simulink model "A1_AAI"  (R2020a)
settings: Solver=FixedStepAuto  StartTime=0.0  StopTime=10  FixedStep=1e-3  RelTol=1e-3  EnableMultiTasking=on
undefined symbols (not defined in the file): D0, D10, D11, D12, D13, D2, D4, D5, D6, D7, D8, D9, PTA0, PTA2, PTB23, PTB9, PTC16, PTC2, PTC3, PTC4, PTD0, PTD1, PTD2, PTD3
libraries: frdmk64flib x16
settings Model: ExtModeTrigDuration=5  Creator=Faisal  LastModifiedBy=Faisal
settings OptimizationCC: EnhancedBackFolding=on  PassReuseOutputArgsAs=Individual arguments  ZeroExternalMemoryAtStartup=off  ZeroInternalMemoryAtStartup=off  MaxStackSize=64  OptimizeBlockOrder=speed  DifferentSizesBufferReuse=on  OptimizationCustomize=off  EfficientTunableParamExpr=on
settings DebuggingCC: ParameterTunabilityLossMsg=error
settings HardwareCC: ProdBitPerPointer=32  ProdBitPerSizeT=32  ProdBitPerPtrDiffT=32  ProdLargestAtomicInteger=Long  ProdLargestAtomicFloat=Double  ProdWordSize=32  ProdHWDeviceType=ARM Compatible->ARM Cortex
settings SFSimCC: MATLABDynamicMemAlloc=off
settings RTWCC: SystemTargetFile=ert.tlc  HardwareBoard=NXP FRDM-K64F  TemplateMakefile=ert_default_tmf  Toolchain=GNU Tools for ARM Embedded Processors
settings CodeAppCC: ForceParamTrailComments=on  IgnoreCustomStorageClasses=off  OperatorAnnotations=on  SimulinkDataObjDesc=on  SFDataObjDesc=on  InsertBlockDesc=on

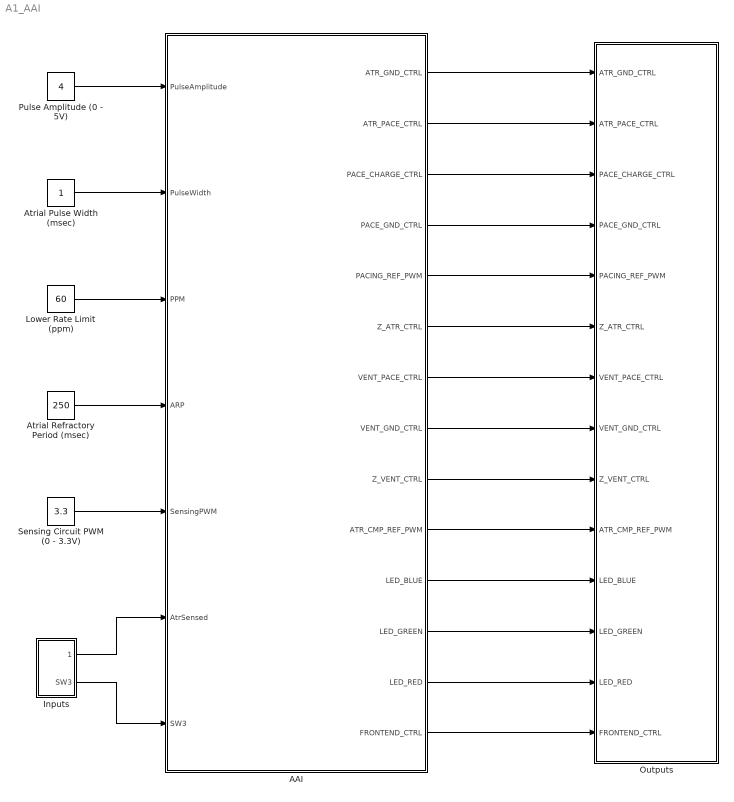
== system A1_AAI ==
  AAI : Stateflow chart  TreatAsAtomicUnit=on
  Atrial Pulse Width (msec) : Constant  OutDataTypeStr=double
  Atrial Refractory Period (msec) : Constant  Value=250  OutDataTypeStr=uint16
  Inputs : Subsystem
  Lower Rate Limit (ppm) : Constant  Value=60  OutDataTypeStr=uint16
  Outputs : Subsystem
  Pulse Amplitude (0 - 5V) : Constant  Value=4  OutDataTypeStr=double
  Sensing Circuit PWM (0 - 3.3V) : Constant  Value=3.3  OutDataTypeStr=double
  wires:
  Pulse Amplitude (0 - 5V)/1 -> AAI/1(PulseAmplitude)
  Atrial Pulse Width (msec)/1 -> AAI/2(PulseWidth)
  Lower Rate Limit (ppm)/1 -> AAI/3(PPM)
  Atrial Refractory Period (msec)/1 -> AAI/4(ARP)
  Sensing Circuit PWM (0 - 3.3V)/1 -> AAI/5(SensingPWM)
  AAI/1(ATR_GND_CTRL) -> Outputs/1(ATR_GND_CTRL)
  AAI/2(ATR_PACE_CTRL) -> Outputs/2(ATR_PACE_CTRL)
  AAI/3(PACE_CHARGE_CTRL) -> Outputs/3(PACE_CHARGE_CTRL)
  AAI/4(PACE_GND_CTRL) -> Outputs/4(PACE_GND_CTRL)
  AAI/5(PACING_REF_PWM) -> Outputs/5(PACING_REF_PWM)
  AAI/6(Z_ATR_CTRL) -> Outputs/6(Z_ATR_CTRL)
  AAI/7(VENT_PACE_CTRL) -> Outputs/7(VENT_PACE_CTRL)
  AAI/8(VENT_GND_CTRL) -> Outputs/8(VENT_GND_CTRL)
  AAI/9(Z_VENT_CTRL) -> Outputs/9(Z_VENT_CTRL)
  AAI/10(ATR_CMP_REF_PWM) -> Outputs/10(ATR_CMP_REF_PWM)
  AAI/11(LED_BLUE) -> Outputs/11(LED_BLUE)
  AAI/12(LED_GREEN) -> Outputs/12(LED_GREEN)
  AAI/13(LED_RED) -> Outputs/13(LED_RED)
  AAI/14(FRONTEND_CTRL) -> Outputs/14(FRONTEND_CTRL)
  Inputs/1(AtrSensed) -> AAI/6(AtrSensed)
  Inputs/2(SW3) -> AAI/7(SW3)

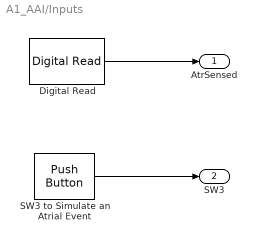
== system A1_AAI/Inputs ==
  Digital Read : frdmk64flib/Digital Read  Whichpin=PTC16 (D0)  SampleTime=-1
  SW3 to Simulate an Atrial Event : frdmk64flib/Push Button  Whichswitch=SW3  SampleTime1=-1
  AtrSensed : Outport
  SW3 : Outport  Port=2
  wires:
  Digital Read/1 -> AtrSensed/1
  SW3 to Simulate an Atrial Event/1 -> SW3/1

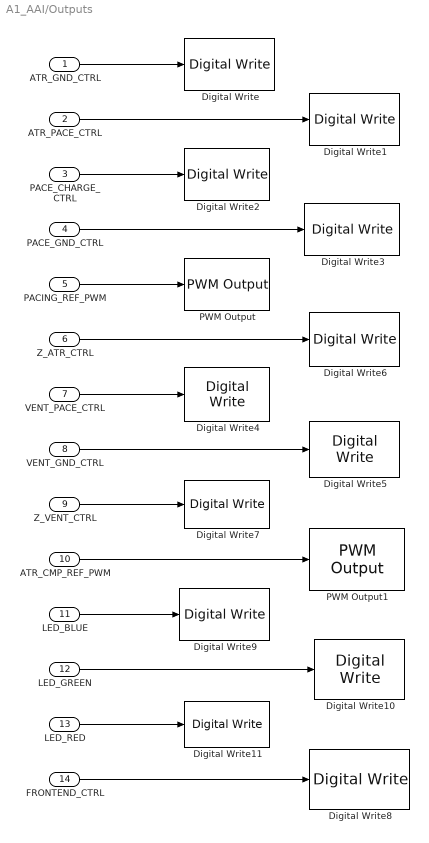
== system A1_AAI/Outputs ==
  ATR_GND_CTRL : Inport
  ATR_PACE_CTRL : Inport  Port=2
  PACE_CHARGE_CTRL : Inport  Port=3
  PACE_GND_CTRL : Inport  Port=4
  PACING_REF_PWM : Inport  Port=5
  Z_ATR_CTRL : Inport  Port=6
  VENT_PACE_CTRL : Inport  Port=7
  VENT_GND_CTRL : Inport  Port=8
  Z_VENT_CTRL : Inport  Port=9
  ATR_CMP_REF_PWM : Inport  Port=10
  LED_BLUE : Inport  Port=11
  LED_GREEN : Inport  Port=12
  LED_RED : Inport  Port=13
  FRONTEND_CTRL : Inport  Port=14
  Digital Write : frdmk64flib/Digital Write  Whichpin=PTD2 (D11)
  Digital Write1 : frdmk64flib/Digital Write  Whichpin=PTA0 (D8)
  Digital Write10 : frdmk64flib/Digital Write  Whichpin=GREEN_LED
  Digital Write11 : frdmk64flib/Digital Write  Whichpin=RED_LED
  Digital Write2 : frdmk64flib/Digital Write  Whichpin=PTB9 (D2)
  Digital Write3 : frdmk64flib/Digital Write  Whichpin=PTD0 (D10)
  Digital Write4 : frdmk64flib/Digital Write  Whichpin=PTC4 (D9)
  Digital Write5 : frdmk64flib/Digital Write  Whichpin=PTD3 (D12)
  Digital Write6 : frdmk64flib/Digital Write  Whichpin=PTB23 (D4)
  Digital Write7 : frdmk64flib/Digital Write  Whichpin=PTC3 (D7)
  Digital Write8 : frdmk64flib/Digital Write  Whichpin=PTD1 (D13)
  Digital Write9 : frdmk64flib/Digital Write  Whichpin=BLUE_LED
  PWM Output : frdmk64flib/PWM Output  Whichpin=PTA2 (D5)  InitialFrequency=2000  InitialDutyCycle=100
  PWM Output1 : frdmk64flib/PWM Output  Whichpin=PTC2 (D6)  InitialFrequency=2000  InitialDutyCycle=0
  wires:
  LED_BLUE/1 -> Digital Write9/1
  VENT_PACE_CTRL/1 -> Digital Write4/1
  Z_ATR_CTRL/1 -> Digital Write6/1
  LED_GREEN/1 -> Digital Write10/1
  PACING_REF_PWM/1 -> PWM Output/1
  PACE_GND_CTRL/1 -> Digital Write3/1
  VENT_GND_CTRL/1 -> Digital Write5/1
  ATR_CMP_REF_PWM/1 -> PWM Output1/1
  FRONTEND_CTRL/1 -> Digital Write8/1
  ATR_PACE_CTRL/1 -> Digital Write1/1
  LED_RED/1 -> Digital Write11/1
  Z_VENT_CTRL/1 -> Digital Write7/1
  ATR_GND_CTRL/1 -> Digital Write/1
  PACE_CHARGE_CTRL/1 -> Digital Write2/1

== stateflow chart A1_AAI/AAI ==
  state Charging_C22
    entry:
    %Charging C22
    ATR_PACE_CTRL=false;
    VENT_PACE_CTRL=false;
    PACING_REF_PWM = 20*PulseAmplitude;
    PACE_CHARGE_CTRL=true;
    %Discharging C21
    PACE_GND_CTRL=true;
    VENT_PACE_CTRL=false;
    Z_ATR_CTRL=false;
    Z_VENT_CTRL=false;
    ATR_GND_CTRL=true;
    VENT_GND_CTRL=false;
    ATR_CMP_REF_PWM = 30.3*SensingPWM;
    FRONTEND_CTRL=true;
    %Turn Red ON
    LED_GREEN=false;
    LED_BLUE=false;
    LED_RED=true;
  state Sense_and_Inhibit
    entry:
    PACING_REF_PWM = 20*PulseAmplitude;
    PACE_CHARGE_CTRL=true;
    %Discharging C21
    PACE_GND_CTRL=true;
    ATR_GND_CTRL=true;
    %Turn Blue ON
    LED_GREEN=false;
    LED_BLUE=true;
    LED_RED=false;
  state Pacing_Atrium
    entry:
    %Discharging C22 into Atrium
    PACE_CHARGE_CTRL=false;
    PACE_GND_CTRL=true;
    ATR_PACE_CTRL=true;
    ATR_GND_CTRL=false;
    Z_ATR_CTRL=false;
    Z_VENT_CTRL=false;
    VENT_GND_CTRL=false;
    VENT_PACE_CTRL=false;
    %Turn Green ON
    LED_GREEN=true;
    LED_BLUE=false;
    LED_RED=false;
  (default) -> Charging_C22
  Pacing_Atrium -> Sense_and_Inhibit : after(PulseWidth,msec)
  Sense_and_Inhibit -> Charging_C22 : after(ARP,msec)
  Charging_C22 -> Sense_and_Inhibit [order 1] : [AtrSensed==true | SW3==true]
  Charging_C22 -> Pacing_Atrium [order 2] : after((60000/PPM)-ARP-PulseWidth,msec)[AtrSensed==false & SW3==false]
  data: ATR_GND_CTRL output boolean; ATR_PACE_CTRL output boolean; PACE_CHARGE_CTRL output boolean; PACE_GND_CTRL output boolean; PACING_REF_PWM output double; Z_ATR_CTRL output boolean; PulseAmplitude input double; PulseWidth input double; PPM input uint16; ARP input uint16; SensingPWM input double; VENT_PACE_CTRL output boolean; VENT_GND_CTRL output boolean; Z_VENT_CTRL output boolean; AtrSensed input boolean; SW3 input boolean; ATR_CMP_REF_PWM output double; LED_BLUE output; LED_GREEN output; LED_RED output; FRONTEND_CTRL output
